simulink library "AEMS_Standard_Library"  (R2016b)
settings: Solver=ode45  StartTime=0.0  StopTime=10.0  RelTol=1e-3
undefined symbols (not defined in the file or in its folder): BkPY, carto, Cbx_extegr, Cbx_lpegrsys, Cbx_portegr, Cnx_bnk_nr_conf, Cnx_cyl_nr_conf, ConfigManagement, configuration_management, Cxx_dcm_io_tmr_end_xxxx, Cxx_dcm_rt_tmr_end, Cxx_DID_xxxx_IO_max, Cxx_DID_xxxx_IO_min, Cxx_egrhsofs, Cxx_vmaniegi, DEM_DEBOUNCE_FREEZE, DEM_DTR_CTL_INVISIBLE, DEM_DTR_CTL_NORMAL, Dem_DtrId2_XXX, Dem_DtrId3_XXX, Dem_DtrId4_XXX, Dem_DtrId5_XXX, Dem_DtrId6_XXX, Dem_DtrId7_XXX, Dem_DtrId8_XXX, Dem_DtrId9_XXX, Dem_DtrId_XXX, Dem_EnableConditionId2_XXX, Dem_EnableConditionId3_XXX, Dem_EnableConditionId4_XXX, Dem_EnableConditionId5_XXX, Dem_EnableConditionId6_XXX, Dem_EnableConditionId7_XXX, Dem_EnableConditionId8_XXX, Dem_EnableConditionId_XXX, Dem_EventId, Dem_EventId2_XXX, Dem_EventId3_XXX, Dem_EventId4_XXX, Dem_EventId5_XXX, Dem_EventId6_XXX, Dem_EventId7_XXX, Dem_EventId8_XXX, Dem_EventId9_XXX, Dem_EventId_Device_Faulttype, Dem_EventId_XXX, DEM_IUMPR_GENERAL_DENOMINATOR, DEM_OPCYC_IGNITION, Dem_RatioId2_XXX, Dem_RatioId3_XXX, Dem_RatioId4_XXX, Dem_RatioId5_XXX, Dem_RatioId6_XXX, Dem_RatioId7_XXX, Dem_RatioId8_XXX, Dem_RatioId_XXX, Dem_StorageConditionId2_XXX, Dem_StorageConditionId3_XXX, Dem_StorageConditionId4_XXX, Dem_StorageConditionId5_XXX ... (+65)
libraries: AEMS_Standard_Library x477, simulink x2
(part 31 of 39)

== system AEMS_Standard_Library/SUB/AEMS_DEM_COUNTER_BASED_DEBOUNCE_THRSHOLD_DYN_8D/AEMS_DEM_COUNTER_BASED_DEBOUNCE_THRSHOLD_DYN_CALL7 ==
  conditionfulfilled : Inport
  prefailed : Inport  Port=2
  prepassed : Inport  Port=3
  DemDebounceBehavior : Inport  Port=4
  failedthreshold : Inport  Port=5
  DemCounterIncrementStepSize : Inport  Port=6
  DemCounterJumpUp : Inport  Port=7
  DemCounterJumpUpValue : Inport  Port=8
  passedthreshold : Inport  Port=9
  DemCounterDecrementStepSize : Inport  Port=10
  DemCounterJumpDown : Inport  Port=11
  DemCounterJumpDownValue : Inport  Port=12
  reseteventdebounce : Inport  Port=13
  Enable : EnablePort
      settings: AttributesFormatString=StatesWhenEnabling = %<StatesWhenEnabling>
  AEMS_DEM_COUNTERBASEDDEBOUNCE : AEMS_Standard_Library/SUB/AEMS_DEM_COUNTERBASEDDEBOUNCE  Tag=[LIB]  eventid=Dem_EventId_Device7_Faulttype
      settings: AttributesFormatString=|
      | %<MaskType>
      | EventId: %<eventid>
  debouncevalue : Outport
      settings: AttributesFormatString=<initial=%<InitialOutput>>\n<whendisabled=%<OutputWhenDisabled>>
  failed : Outport  Port=2
      settings: AttributesFormatString=<initial=%<InitialOutput>>\n<whendisabled=%<OutputWhenDisabled>>
  passed : Outport  Port=3
      settings: AttributesFormatString=<initial=%<InitialOutput>>\n<whendisabled=%<OutputWhenDisabled>>
  wires:
  DemCounterJumpDownValue/1 -> AEMS_DEM_COUNTERBASEDDEBOUNCE/13
  DemCounterDecrementStepSize/1 -> AEMS_DEM_COUNTERBASEDDEBOUNCE/11
  DemCounterJumpUp/1 -> AEMS_DEM_COUNTERBASEDDEBOUNCE/8
  DemCounterIncrementStepSize/1 -> AEMS_DEM_COUNTERBASEDDEBOUNCE/7
  DemDebounceBehavior/1 -> AEMS_DEM_COUNTERBASEDDEBOUNCE/5
  DemCounterJumpDown/1 -> AEMS_DEM_COUNTERBASEDDEBOUNCE/12
  failedthreshold/1 -> AEMS_DEM_COUNTERBASEDDEBOUNCE/6
  passedthreshold/1 -> AEMS_DEM_COUNTERBASEDDEBOUNCE/10
  DemCounterJumpUpValue/1 -> AEMS_DEM_COUNTERBASEDDEBOUNCE/9
  reseteventdebounce/1 -> AEMS_DEM_COUNTERBASEDDEBOUNCE/4
  AEMS_DEM_COUNTERBASEDDEBOUNCE/3 -> passed/1
  AEMS_DEM_COUNTERBASEDDEBOUNCE/2 -> failed/1
  AEMS_DEM_COUNTERBASEDDEBOUNCE/1 -> debouncevalue/1
  prefailed/1 -> AEMS_DEM_COUNTERBASEDDEBOUNCE/2
  prepassed/1 -> AEMS_DEM_COUNTERBASEDDEBOUNCE/3
  conditionfulfilled/1 -> AEMS_DEM_COUNTERBASEDDEBOUNCE/1

== system AEMS_Standard_Library/SUB/AEMS_DEM_COUNTER_BASED_DEBOUNCE_THRSHOLD_DYN_8D/AEMS_DEM_COUNTER_BASED_DEBOUNCE_THRSHOLD_DYN_CALL8 ==
  conditionfulfilled : Inport
  prefailed : Inport  Port=2
  prepassed : Inport  Port=3
  DemDebounceBehavior : Inport  Port=4
  failedthreshold : Inport  Port=5
  DemCounterIncrementStepSize : Inport  Port=6
  DemCounterJumpUp : Inport  Port=7
  DemCounterJumpUpValue : Inport  Port=8
  passedthreshold : Inport  Port=9
  DemCounterDecrementStepSize : Inport  Port=10
  DemCounterJumpDown : Inport  Port=11
  DemCounterJumpDownValue : Inport  Port=12
  reseteventdebounce : Inport  Port=13
  Enable : EnablePort
      settings: AttributesFormatString=StatesWhenEnabling = %<StatesWhenEnabling>
  AEMS_DEM_COUNTERBASEDDEBOUNCE : AEMS_Standard_Library/SUB/AEMS_DEM_COUNTERBASEDDEBOUNCE  Tag=[LIB]  eventid=Dem_EventId_Device8_Faulttype
      settings: AttributesFormatString=|
      | %<MaskType>
      | EventId: %<eventid>
  debouncevalue : Outport
      settings: AttributesFormatString=<initial=%<InitialOutput>>\n<whendisabled=%<OutputWhenDisabled>>
  failed : Outport  Port=2
      settings: AttributesFormatString=<initial=%<InitialOutput>>\n<whendisabled=%<OutputWhenDisabled>>
  passed : Outport  Port=3
      settings: AttributesFormatString=<initial=%<InitialOutput>>\n<whendisabled=%<OutputWhenDisabled>>
  wires:
  DemCounterJumpUp/1 -> AEMS_DEM_COUNTERBASEDDEBOUNCE/8
  failedthreshold/1 -> AEMS_DEM_COUNTERBASEDDEBOUNCE/6
  DemCounterJumpDown/1 -> AEMS_DEM_COUNTERBASEDDEBOUNCE/12
  passedthreshold/1 -> AEMS_DEM_COUNTERBASEDDEBOUNCE/10
  DemCounterIncrementStepSize/1 -> AEMS_DEM_COUNTERBASEDDEBOUNCE/7
  DemDebounceBehavior/1 -> AEMS_DEM_COUNTERBASEDDEBOUNCE/5
  DemCounterDecrementStepSize/1 -> AEMS_DEM_COUNTERBASEDDEBOUNCE/11
  DemCounterJumpDownValue/1 -> AEMS_DEM_COUNTERBASEDDEBOUNCE/13
  DemCounterJumpUpValue/1 -> AEMS_DEM_COUNTERBASEDDEBOUNCE/9
  reseteventdebounce/1 -> AEMS_DEM_COUNTERBASEDDEBOUNCE/4
  conditionfulfilled/1 -> AEMS_DEM_COUNTERBASEDDEBOUNCE/1
  prepassed/1 -> AEMS_DEM_COUNTERBASEDDEBOUNCE/3
  prefailed/1 -> AEMS_DEM_COUNTERBASEDDEBOUNCE/2
  AEMS_DEM_COUNTERBASEDDEBOUNCE/1 -> debouncevalue/1
  AEMS_DEM_COUNTERBASEDDEBOUNCE/2 -> failed/1
  AEMS_DEM_COUNTERBASEDDEBOUNCE/3 -> passed/1

== system AEMS_Standard_Library/SUB/AEMS_DEM_REP_IUMPR_1D/Dem_RepIUMPRDenLock_call1 ==
  denlock_call1 : EnablePort
      settings: AttributesFormatString=<states=%<StatesWhenEnabling>>
  AEMS_DEM_REPIUMPRDENLOCK1 : AEMS_Standard_Library/SUB/AEMS_DEM_REPIUMPRDENLOCK  Tag=[LIB]
      settings: AttributesFormatString=%<MaskType>
  RatioId_block1 : Constant  Value=Dem_RatioId_XXX  OutDataTypeStr=uint16
  wires:
  RatioId_block1/1 -> AEMS_DEM_REPIUMPRDENLOCK1/1  "ratioid"

== system AEMS_Standard_Library/SUB/AEMS_DEM_REP_IUMPR_1D/Dem_RepIUMPRDenRelease_call1 ==
  denrelease_call1 : EnablePort
      settings: AttributesFormatString=<states=%<StatesWhenEnabling>>
  AEMS_DEM_REPIUMPRDENRELEASE1 : AEMS_Standard_Library/SUB/AEMS_DEM_REPIUMPRDENRELEASE  Tag=[LIB]
      settings: AttributesFormatString=%<MaskType>
  RatioId_block1 : Constant  Value=Dem_RatioId_XXX  OutDataTypeStr=uint16
  wires:
  RatioId_block1/1 -> AEMS_DEM_REPIUMPRDENRELEASE1/1  "ratioid"

== system AEMS_Standard_Library/SUB/AEMS_DEM_REP_IUMPR_1D/Dem_RepIUMPRFaultDetect_call1 ==
  faultdetect_call1 : EnablePort
      settings: AttributesFormatString=<states=%<StatesWhenEnabling>>
  AEMS_DEM_REPIUMPRFAULTDETECT1 : AEMS_Standard_Library/SUB/AEMS_DEM_REPIUMPRFAULTDETECT  Tag=[LIB]
      settings: AttributesFormatString=%<MaskType>
  RatioId_block1 : Constant  Value=Dem_RatioId_XXX  OutDataTypeStr=uint16
  wires:
  RatioId_block1/1 -> AEMS_DEM_REPIUMPRFAULTDETECT1/1  "ratioid"

== system AEMS_Standard_Library/SUB/AEMS_DEM_REP_IUMPR_2D/Dem_RepIUMPRDenLock_Call1 ==
  denlock_call1 : EnablePort
      settings: AttributesFormatString=<states=%<StatesWhenEnabling>>
  AEMS_DEM_REPIUMPRDENLOCK1 : AEMS_Standard_Library/SUB/AEMS_DEM_REPIUMPRDENLOCK
      settings: AttributesFormatString=%<MaskType>
  RatioId_block1 : Constant  Value=Dem_RatioId_XXX  OutDataTypeStr=uint16
  wires:
  RatioId_block1/1 -> AEMS_DEM_REPIUMPRDENLOCK1/1  "ratioid1"

== system AEMS_Standard_Library/SUB/AEMS_DEM_REP_IUMPR_2D/Dem_RepIUMPRDenLock_Call2 ==
  denlock_call2 : EnablePort
      settings: AttributesFormatString=<states=%<StatesWhenEnabling>>
  AEMS_DEM_REPIUMPRDENLOCK2 : AEMS_Standard_Library/SUB/AEMS_DEM_REPIUMPRDENLOCK
      settings: AttributesFormatString=%<MaskType>
  RatioId_block2 : Constant  Value=Dem_RatioId2_XXX  OutDataTypeStr=uint16
  wires:
  RatioId_block2/1 -> AEMS_DEM_REPIUMPRDENLOCK2/1  "ratioid2"

== system AEMS_Standard_Library/SUB/AEMS_DEM_REP_IUMPR_2D/Dem_RepIUMPRDenRelease_Call1 ==
  denrelease_call1 : EnablePort
      settings: AttributesFormatString=<states=%<StatesWhenEnabling>>
  AEMS_DEM_REPIUMPRDENRELEASE1 : AEMS_Standard_Library/SUB/AEMS_DEM_REPIUMPRDENRELEASE
      settings: AttributesFormatString=%<MaskType>
  RatioId_block1 : Constant  Value=Dem_RatioId_XXX  OutDataTypeStr=uint16
  wires:
  RatioId_block1/1 -> AEMS_DEM_REPIUMPRDENRELEASE1/1  "ratioid1"

== system AEMS_Standard_Library/SUB/AEMS_DEM_REP_IUMPR_2D/Dem_RepIUMPRDenRelease_Call2 ==
  denrelease_call2 : EnablePort
      settings: AttributesFormatString=<states=%<StatesWhenEnabling>>
  AEMS_DEM_REPIUMPRDENRELEASE2 : AEMS_Standard_Library/SUB/AEMS_DEM_REPIUMPRDENRELEASE
      settings: AttributesFormatString=%<MaskType>
  RatioId_block2 : Constant  Value=Dem_RatioId2_XXX  OutDataTypeStr=uint16
  wires:
  RatioId_block2/1 -> AEMS_DEM_REPIUMPRDENRELEASE2/1  "ratioid2"

== system AEMS_Standard_Library/SUB/AEMS_DEM_REP_IUMPR_2D/Dem_RepIUMPRFaultDetect_Call1 ==
  faultdetect_call1 : EnablePort
      settings: AttributesFormatString=<states=%<StatesWhenEnabling>>
  AEMS_DEM_REPIUMPRFAULTDETECT1 : AEMS_Standard_Library/SUB/AEMS_DEM_REPIUMPRFAULTDETECT
      settings: AttributesFormatString=%<MaskType>
  RatioId_block1 : Constant  Value=Dem_RatioId_XXX  OutDataTypeStr=uint16
  wires:
  RatioId_block1/1 -> AEMS_DEM_REPIUMPRFAULTDETECT1/1  "ratioid1"

== system AEMS_Standard_Library/SUB/AEMS_DEM_REP_IUMPR_2D/Dem_RepIUMPRFaultDetect_Call2 ==
  faultdetect_call2 : EnablePort
      settings: AttributesFormatString=<states=%<StatesWhenEnabling>>
  AEMS_DEM_REPIUMPRFAULTDETECT2 : AEMS_Standard_Library/SUB/AEMS_DEM_REPIUMPRFAULTDETECT
      settings: AttributesFormatString=%<MaskType>
  RatioId_block2 : Constant  Value=Dem_RatioId2_XXX  OutDataTypeStr=uint16
  wires:
  RatioId_block2/1 -> AEMS_DEM_REPIUMPRFAULTDETECT2/1  "ratioid2"

== system AEMS_Standard_Library/SUB/AEMS_DEM_REP_IUMPR_8D/Dem_RepIUMPRDenLock_Call1 ==
  denlock_call1 : EnablePort
      settings: AttributesFormatString=<states=%<StatesWhenEnabling>>
  AEMS_DEM_REPIUMPRDENLOCK1 : AEMS_Standard_Library/SUB/AEMS_DEM_REPIUMPRDENLOCK  Tag=[LIB]
      settings: AttributesFormatString=%<MaskType>
  RatioId_block1 : Constant  Value=Dem_RatioId_XXX  OutDataTypeStr=uint16
  wires:
  RatioId_block1/1 -> AEMS_DEM_REPIUMPRDENLOCK1/1  "ratioid1"

== system AEMS_Standard_Library/SUB/AEMS_DEM_REP_IUMPR_8D/Dem_RepIUMPRDenLock_Call2 ==
  denlock_call2 : EnablePort
      settings: AttributesFormatString=<states=%<StatesWhenEnabling>>
  AEMS_DEM_REPIUMPRDENLOCK2 : AEMS_Standard_Library/SUB/AEMS_DEM_REPIUMPRDENLOCK  Tag=[LIB]
      settings: AttributesFormatString=%<MaskType>
  RatioId_block2 : Constant  Value=Dem_RatioId2_XXX  OutDataTypeStr=uint16
  wires:
  RatioId_block2/1 -> AEMS_DEM_REPIUMPRDENLOCK2/1  "ratioid2"

== system AEMS_Standard_Library/SUB/AEMS_DEM_REP_IUMPR_8D/Dem_RepIUMPRDenLock_Call3 ==
  denlock_call3 : EnablePort
      settings: AttributesFormatString=<states=%<StatesWhenEnabling>>
  AEMS_DEM_REPIUMPRDENLOCK3 : AEMS_Standard_Library/SUB/AEMS_DEM_REPIUMPRDENLOCK  Tag=[LIB]
      settings: AttributesFormatString=%<MaskType>
  RatioId_block3 : Constant  Value=Dem_RatioId3_XXX  OutDataTypeStr=uint16
  wires:
  RatioId_block3/1 -> AEMS_DEM_REPIUMPRDENLOCK3/1  "ratioid3"

== system AEMS_Standard_Library/SUB/AEMS_DEM_REP_IUMPR_8D/Dem_RepIUMPRDenLock_Call4 ==
  denlock_call4 : EnablePort
      settings: AttributesFormatString=<states=%<StatesWhenEnabling>>
  AEMS_DEM_REPIUMPRDENLOCK4 : AEMS_Standard_Library/SUB/AEMS_DEM_REPIUMPRDENLOCK  Tag=[LIB]
      settings: AttributesFormatString=%<MaskType>
  RatioId_block4 : Constant  Value=Dem_RatioId4_XXX  OutDataTypeStr=uint16
  wires:
  RatioId_block4/1 -> AEMS_DEM_REPIUMPRDENLOCK4/1  "ratioid4"

== system AEMS_Standard_Library/SUB/AEMS_DEM_REP_IUMPR_8D/Dem_RepIUMPRDenLock_Call5 ==
  denlock_call5 : EnablePort
      settings: AttributesFormatString=<states=%<StatesWhenEnabling>>
  AEMS_DEM_REPIUMPRDENLOCK5 : AEMS_Standard_Library/SUB/AEMS_DEM_REPIUMPRDENLOCK  Tag=[LIB]
      settings: AttributesFormatString=%<MaskType>
  RatioId_block5 : Constant  Value=Dem_RatioId5_XXX  OutDataTypeStr=uint16
  wires:
  RatioId_block5/1 -> AEMS_DEM_REPIUMPRDENLOCK5/1  "ratioid5"

== system AEMS_Standard_Library/SUB/AEMS_DEM_REP_IUMPR_8D/Dem_RepIUMPRDenLock_Call6 ==
  denlock_call6 : EnablePort
      settings: AttributesFormatString=<states=%<StatesWhenEnabling>>
  AEMS_DEM_REPIUMPRDENLOCK6 : AEMS_Standard_Library/SUB/AEMS_DEM_REPIUMPRDENLOCK  Tag=[LIB]
      settings: AttributesFormatString=%<MaskType>
  RatioId_block6 : Constant  Value=Dem_RatioId6_XXX  OutDataTypeStr=uint16
  wires:
  RatioId_block6/1 -> AEMS_DEM_REPIUMPRDENLOCK6/1  "ratioid6"

== system AEMS_Standard_Library/SUB/AEMS_DEM_REP_IUMPR_8D/Dem_RepIUMPRDenLock_Call7 ==
  denlock_call7 : EnablePort
      settings: AttributesFormatString=<states=%<StatesWhenEnabling>>
  AEMS_DEM_REPIUMPRDENLOCK7 : AEMS_Standard_Library/SUB/AEMS_DEM_REPIUMPRDENLOCK  Tag=[LIB]
      settings: AttributesFormatString=%<MaskType>
  RatioId_block7 : Constant  Value=Dem_RatioId7_XXX  OutDataTypeStr=uint16
  wires:
  RatioId_block7/1 -> AEMS_DEM_REPIUMPRDENLOCK7/1  "ratioid7"

== system AEMS_Standard_Library/SUB/AEMS_DEM_REP_IUMPR_8D/Dem_RepIUMPRDenLock_Call8 ==
  denlock_call8 : EnablePort
      settings: AttributesFormatString=<states=%<StatesWhenEnabling>>
  AEMS_DEM_REPIUMPRDENLOCK8 : AEMS_Standard_Library/SUB/AEMS_DEM_REPIUMPRDENLOCK  Tag=[LIB]
      settings: AttributesFormatString=%<MaskType>
  RatioId_block8 : Constant  Value=Dem_RatioId8_XXX  OutDataTypeStr=uint16
  wires:
  RatioId_block8/1 -> AEMS_DEM_REPIUMPRDENLOCK8/1  "ratioid8"

== system AEMS_Standard_Library/SUB/AEMS_DEM_REP_IUMPR_8D/Dem_RepIUMPRDenRelease_Call1 ==
  denrelease_call1 : EnablePort
      settings: AttributesFormatString=<states=%<StatesWhenEnabling>>
  AEMS_DEM_REPIUMPRDENRELEASE1 : AEMS_Standard_Library/SUB/AEMS_DEM_REPIUMPRDENRELEASE  Tag=[LIB]
      settings: AttributesFormatString=%<MaskType>
  RatioId_block1 : Constant  Value=Dem_RatioId_XXX  OutDataTypeStr=uint16
  wires:
  RatioId_block1/1 -> AEMS_DEM_REPIUMPRDENRELEASE1/1  "ratioid1"

== system AEMS_Standard_Library/SUB/AEMS_DEM_REP_IUMPR_8D/Dem_RepIUMPRDenRelease_Call2 ==
  denrelease_call2 : EnablePort
      settings: AttributesFormatString=<states=%<StatesWhenEnabling>>
  AEMS_DEM_REPIUMPRDENRELEASE2 : AEMS_Standard_Library/SUB/AEMS_DEM_REPIUMPRDENRELEASE  Tag=[LIB]
      settings: AttributesFormatString=%<MaskType>
  RatioId_block2 : Constant  Value=Dem_RatioId2_XXX  OutDataTypeStr=uint16
  wires:
  RatioId_block2/1 -> AEMS_DEM_REPIUMPRDENRELEASE2/1  "ratioid2"

== system AEMS_Standard_Library/SUB/AEMS_DEM_REP_IUMPR_8D/Dem_RepIUMPRDenRelease_Call3 ==
  denrelease_call3 : EnablePort
      settings: AttributesFormatString=<states=%<StatesWhenEnabling>>
  AEMS_DEM_REPIUMPRDENRELEASE3 : AEMS_Standard_Library/SUB/AEMS_DEM_REPIUMPRDENRELEASE  Tag=[LIB]
      settings: AttributesFormatString=%<MaskType>
  RatioId_block3 : Constant  Value=Dem_RatioId3_XXX  OutDataTypeStr=uint16
  wires:
  RatioId_block3/1 -> AEMS_DEM_REPIUMPRDENRELEASE3/1  "ratioid3"

== system AEMS_Standard_Library/SUB/AEMS_DEM_REP_IUMPR_8D/Dem_RepIUMPRDenRelease_Call4 ==
  denrelease_call4 : EnablePort
      settings: AttributesFormatString=<states=%<StatesWhenEnabling>>
  AEMS_DEM_REPIUMPRDENRELEASE4 : AEMS_Standard_Library/SUB/AEMS_DEM_REPIUMPRDENRELEASE  Tag=[LIB]
      settings: AttributesFormatString=%<MaskType>
  RatioId_block4 : Constant  Value=Dem_RatioId4_XXX  OutDataTypeStr=uint16
  wires:
  RatioId_block4/1 -> AEMS_DEM_REPIUMPRDENRELEASE4/1  "ratioid4"

== system AEMS_Standard_Library/SUB/AEMS_DEM_REP_IUMPR_8D/Dem_RepIUMPRDenRelease_Call5 ==
  denrelease_call5 : EnablePort
      settings: AttributesFormatString=<states=%<StatesWhenEnabling>>
  AEMS_DEM_REPIUMPRDENRELEASE5 : AEMS_Standard_Library/SUB/AEMS_DEM_REPIUMPRDENRELEASE  Tag=[LIB]
      settings: AttributesFormatString=%<MaskType>
  RatioId_block5 : Constant  Value=Dem_RatioId5_XXX  OutDataTypeStr=uint16
  wires:
  RatioId_block5/1 -> AEMS_DEM_REPIUMPRDENRELEASE5/1  "ratioid5"

== system AEMS_Standard_Library/SUB/AEMS_DEM_REP_IUMPR_8D/Dem_RepIUMPRDenRelease_Call6 ==
  denrelease_call6 : EnablePort
      settings: AttributesFormatString=<states=%<StatesWhenEnabling>>
  AEMS_DEM_REPIUMPRDENRELEASE6 : AEMS_Standard_Library/SUB/AEMS_DEM_REPIUMPRDENRELEASE  Tag=[LIB]
      settings: AttributesFormatString=%<MaskType>
  RatioId_block6 : Constant  Value=Dem_RatioId6_XXX  OutDataTypeStr=uint16
  wires:
  RatioId_block6/1 -> AEMS_DEM_REPIUMPRDENRELEASE6/1  "ratioid6"

== system AEMS_Standard_Library/SUB/AEMS_DEM_REP_IUMPR_8D/Dem_RepIUMPRDenRelease_Call7 ==
  denrelease_call7 : EnablePort
      settings: AttributesFormatString=<states=%<StatesWhenEnabling>>
  AEMS_DEM_REPIUMPRDENRELEASE7 : AEMS_Standard_Library/SUB/AEMS_DEM_REPIUMPRDENRELEASE  Tag=[LIB]
      settings: AttributesFormatString=%<MaskType>
  RatioId_block7 : Constant  Value=Dem_RatioId7_XXX  OutDataTypeStr=uint16
  wires:
  RatioId_block7/1 -> AEMS_DEM_REPIUMPRDENRELEASE7/1  "ratioid7"

== system AEMS_Standard_Library/SUB/AEMS_DEM_REP_IUMPR_8D/Dem_RepIUMPRDenRelease_Call8 ==
  denrelease_call8 : EnablePort
      settings: AttributesFormatString=<states=%<StatesWhenEnabling>>
  AEMS_DEM_REPIUMPRDENRELEASE8 : AEMS_Standard_Library/SUB/AEMS_DEM_REPIUMPRDENRELEASE  Tag=[LIB]
      settings: AttributesFormatString=%<MaskType>
  RatioId_block8 : Constant  Value=Dem_RatioId8_XXX  OutDataTypeStr=uint16
  wires:
  RatioId_block8/1 -> AEMS_DEM_REPIUMPRDENRELEASE8/1  "ratioid8"

== system AEMS_Standard_Library/SUB/AEMS_DEM_REP_IUMPR_8D/Dem_RepIUMPRFaultDetect_Call1 ==
  faultdetect_call1 : EnablePort
      settings: AttributesFormatString=<states=%<StatesWhenEnabling>>
  AEMS_DEM_REPIUMPRFAULTDETECT1 : AEMS_Standard_Library/SUB/AEMS_DEM_REPIUMPRFAULTDETECT  Tag=[LIB]
      settings: AttributesFormatString=%<MaskType>
  RatioId_block1 : Constant  Value=Dem_RatioId_XXX  OutDataTypeStr=uint16
  wires:
  RatioId_block1/1 -> AEMS_DEM_REPIUMPRFAULTDETECT1/1  "ratioid1"

== system AEMS_Standard_Library/SUB/AEMS_DEM_REP_IUMPR_8D/Dem_RepIUMPRFaultDetect_Call2 ==
  faultdetect_call2 : EnablePort
      settings: AttributesFormatString=<states=%<StatesWhenEnabling>>
  AEMS_DEM_REPIUMPRFAULTDETECT2 : AEMS_Standard_Library/SUB/AEMS_DEM_REPIUMPRFAULTDETECT  Tag=[LIB]
      settings: AttributesFormatString=%<MaskType>
  RatioId_block2 : Constant  Value=Dem_RatioId2_XXX  OutDataTypeStr=uint16
  wires:
  RatioId_block2/1 -> AEMS_DEM_REPIUMPRFAULTDETECT2/1  "ratioid2"

== system AEMS_Standard_Library/SUB/AEMS_DEM_REP_IUMPR_8D/Dem_RepIUMPRFaultDetect_Call3 ==
  faultdetect_call3 : EnablePort
      settings: AttributesFormatString=<states=%<StatesWhenEnabling>>
  AEMS_DEM_REPIUMPRFAULTDETECT3 : AEMS_Standard_Library/SUB/AEMS_DEM_REPIUMPRFAULTDETECT  Tag=[LIB]
      settings: AttributesFormatString=%<MaskType>
  RatioId_block3 : Constant  Value=Dem_RatioId3_XXX  OutDataTypeStr=uint16
  wires:
  RatioId_block3/1 -> AEMS_DEM_REPIUMPRFAULTDETECT3/1  "ratioid3"

== system AEMS_Standard_Library/SUB/AEMS_DEM_REP_IUMPR_8D/Dem_RepIUMPRFaultDetect_Call4 ==
  faultdetect_call4 : EnablePort
      settings: AttributesFormatString=<states=%<StatesWhenEnabling>>
  AEMS_DEM_REPIUMPRFAULTDETECT4 : AEMS_Standard_Library/SUB/AEMS_DEM_REPIUMPRFAULTDETECT  Tag=[LIB]
      settings: AttributesFormatString=%<MaskType>
  RatioId_block4 : Constant  Value=Dem_RatioId4_XXX  OutDataTypeStr=uint16
  wires:
  RatioId_block4/1 -> AEMS_DEM_REPIUMPRFAULTDETECT4/1  "ratioid4"

== system AEMS_Standard_Library/SUB/AEMS_DEM_REP_IUMPR_8D/Dem_RepIUMPRFaultDetect_Call5 ==
  faultdetect_call5 : EnablePort
      settings: AttributesFormatString=<states=%<StatesWhenEnabling>>
  AEMS_DEM_REPIUMPRFAULTDETECT5 : AEMS_Standard_Library/SUB/AEMS_DEM_REPIUMPRFAULTDETECT  Tag=[LIB]
      settings: AttributesFormatString=%<MaskType>
  RatioId_block5 : Constant  Value=Dem_RatioId5_XXX  OutDataTypeStr=uint16
  wires:
  RatioId_block5/1 -> AEMS_DEM_REPIUMPRFAULTDETECT5/1  "ratioid5"

== system AEMS_Standard_Library/SUB/AEMS_DEM_REP_IUMPR_8D/Dem_RepIUMPRFaultDetect_Call6 ==
  faultdetect_call6 : EnablePort
      settings: AttributesFormatString=<states=%<StatesWhenEnabling>>
  AEMS_DEM_REPIUMPRFAULTDETECT6 : AEMS_Standard_Library/SUB/AEMS_DEM_REPIUMPRFAULTDETECT  Tag=[LIB]
      settings: AttributesFormatString=%<MaskType>
  RatioId_block6 : Constant  Value=Dem_RatioId6_XXX  OutDataTypeStr=uint16
  wires:
  RatioId_block6/1 -> AEMS_DEM_REPIUMPRFAULTDETECT6/1  "ratioid6"

== system AEMS_Standard_Library/SUB/AEMS_DEM_REP_IUMPR_8D/Dem_RepIUMPRFaultDetect_Call7 ==
  faultdetect_call7 : EnablePort
      settings: AttributesFormatString=<states=%<StatesWhenEnabling>>
  AEMS_DEM_REPIUMPRFAULTDETECT7 : AEMS_Standard_Library/SUB/AEMS_DEM_REPIUMPRFAULTDETECT  Tag=[LIB]
      settings: AttributesFormatString=%<MaskType>
  RatioId_block7 : Constant  Value=Dem_RatioId7_XXX  OutDataTypeStr=uint16
  wires:
  RatioId_block7/1 -> AEMS_DEM_REPIUMPRFAULTDETECT7/1  "ratioid7"

== system AEMS_Standard_Library/SUB/AEMS_DEM_REP_IUMPR_8D/Dem_RepIUMPRFaultDetect_Call8 ==
  faultdetect_call8 : EnablePort
      settings: AttributesFormatString=<states=%<StatesWhenEnabling>>
  AEMS_DEM_REPIUMPRFAULTDETECT8 : AEMS_Standard_Library/SUB/AEMS_DEM_REPIUMPRFAULTDETECT  Tag=[LIB]
      settings: AttributesFormatString=%<MaskType>
  RatioId_block8 : Constant  Value=Dem_RatioId8_XXX  OutDataTypeStr=uint16
  wires:
  RatioId_block8/1 -> AEMS_DEM_REPIUMPRFAULTDETECT8/1  "ratioid8"

== system AEMS_Standard_Library/SUB/AEMS_DEM_REP_IUMPR_DEN_RELEASE_1D/Dem_RepIUMPRDenRelease_call ==
  denrelease_call : EnablePort
      settings: AttributesFormatString=<states=%<StatesWhenEnabling>>
  AEMS_DEM_REPIUMPRDENRELEASE : AEMS_Standard_Library/SUB/AEMS_DEM_REPIUMPRDENRELEASE  Tag=[LIB]
      settings: AttributesFormatString=%<MaskType>
  RatioId_block1 : Constant  Value=Dem_RatioId_XXX  OutDataTypeStr=uint16
  wires:
  RatioId_block1/1 -> AEMS_DEM_REPIUMPRDENRELEASE/1  "ratioid"

== system AEMS_Standard_Library/SUB/AEMS_DEM_REP_IUMPR_DEN_RELEASE_2D/Dem_RepIUMPRDenRelease_call1 ==
  denrelease_call1 : EnablePort
      settings: AttributesFormatString=<states=%<StatesWhenEnabling>>
  AEMS_DEM_REPIUMPRDENRELEASE : AEMS_Standard_Library/SUB/AEMS_DEM_REPIUMPRDENRELEASE  Tag=[LIB]
      settings: AttributesFormatString=%<MaskType>
  RatioId_block1 : Constant  Value=Dem_RatioId_XXX  OutDataTypeStr=uint16
  wires:
  RatioId_block1/1 -> AEMS_DEM_REPIUMPRDENRELEASE/1  "ratioid1"

== system AEMS_Standard_Library/SUB/AEMS_DEM_REP_IUMPR_DEN_RELEASE_2D/Dem_RepIUMPRDenRelease_call2 ==
  denrelease_call2 : EnablePort
      settings: AttributesFormatString=<states=%<StatesWhenEnabling>>
  AEMS_DEM_REPIUMPRDENRELEASE : AEMS_Standard_Library/SUB/AEMS_DEM_REPIUMPRDENRELEASE  Tag=[LIB]
      settings: AttributesFormatString=%<MaskType>
  RatioId_block2 : Constant  Value=Dem_RatioId2_XXX  OutDataTypeStr=uint16
  wires:
  RatioId_block2/1 -> AEMS_DEM_REPIUMPRDENRELEASE/1  "ratioid2"

== system AEMS_Standard_Library/SUB/AEMS_DEM_REP_IUMPR_DEN_RELEASE_8D/Dem_RepIUMPRDenRelease_call1 ==
  denrelease_call1 : EnablePort
      settings: AttributesFormatString=<states=%<StatesWhenEnabling>>
  AEMS_DEM_REPIUMPRDENRELEASE : AEMS_Standard_Library/SUB/AEMS_DEM_REPIUMPRDENRELEASE  Tag=[LIB]
      settings: AttributesFormatString=%<MaskType>
  RatioId_block1 : Constant  Value=Dem_RatioId_XXX  OutDataTypeStr=uint16
  wires:
  RatioId_block1/1 -> AEMS_DEM_REPIUMPRDENRELEASE/1  "ratioid1"

== system AEMS_Standard_Library/SUB/AEMS_DEM_REP_IUMPR_DEN_RELEASE_8D/Dem_RepIUMPRDenRelease_call2 ==
  denrelease_call2 : EnablePort
      settings: AttributesFormatString=<states=%<StatesWhenEnabling>>
  AEMS_DEM_REPIUMPRDENRELEASE : AEMS_Standard_Library/SUB/AEMS_DEM_REPIUMPRDENRELEASE  Tag=[LIB]
      settings: AttributesFormatString=%<MaskType>
  RatioId_block2 : Constant  Value=Dem_RatioId2_XXX  OutDataTypeStr=uint16
  wires:
  RatioId_block2/1 -> AEMS_DEM_REPIUMPRDENRELEASE/1  "ratioid2"

== system AEMS_Standard_Library/SUB/AEMS_DEM_REP_IUMPR_DEN_RELEASE_8D/Dem_RepIUMPRDenRelease_call3 ==
  denrelease_call3 : EnablePort
      settings: AttributesFormatString=<states=%<StatesWhenEnabling>>
  AEMS_DEM_REPIUMPRDENRELEASE : AEMS_Standard_Library/SUB/AEMS_DEM_REPIUMPRDENRELEASE  Tag=[LIB]
      settings: AttributesFormatString=%<MaskType>
  RatioId_block3 : Constant  Value=Dem_RatioId3_XXX  OutDataTypeStr=uint16
  wires:
  RatioId_block3/1 -> AEMS_DEM_REPIUMPRDENRELEASE/1  "ratioid3"

== system AEMS_Standard_Library/SUB/AEMS_DEM_REP_IUMPR_DEN_RELEASE_8D/Dem_RepIUMPRDenRelease_call4 ==
  denrelease_call4 : EnablePort
      settings: AttributesFormatString=<states=%<StatesWhenEnabling>>
  AEMS_DEM_REPIUMPRDENRELEASE : AEMS_Standard_Library/SUB/AEMS_DEM_REPIUMPRDENRELEASE  Tag=[LIB]
      settings: AttributesFormatString=%<MaskType>
  RatioId_block4 : Constant  Value=Dem_RatioId4_XXX  OutDataTypeStr=uint16
  wires:
  RatioId_block4/1 -> AEMS_DEM_REPIUMPRDENRELEASE/1  "ratioid4"

== system AEMS_Standard_Library/SUB/AEMS_DEM_REP_IUMPR_DEN_RELEASE_8D/Dem_RepIUMPRDenRelease_call5 ==
  denrelease_call5 : EnablePort
      settings: AttributesFormatString=<states=%<StatesWhenEnabling>>
  AEMS_DEM_REPIUMPRDENRELEASE : AEMS_Standard_Library/SUB/AEMS_DEM_REPIUMPRDENRELEASE  Tag=[LIB]
      settings: AttributesFormatString=%<MaskType>
  RatioId_block5 : Constant  Value=Dem_RatioId5_XXX  OutDataTypeStr=uint16
  wires:
  RatioId_block5/1 -> AEMS_DEM_REPIUMPRDENRELEASE/1  "ratioid5"

== system AEMS_Standard_Library/SUB/AEMS_DEM_REP_IUMPR_DEN_RELEASE_8D/Dem_RepIUMPRDenRelease_call6 ==
  denrelease_call6 : EnablePort
      settings: AttributesFormatString=<states=%<StatesWhenEnabling>>
  AEMS_DEM_REPIUMPRDENRELEASE : AEMS_Standard_Library/SUB/AEMS_DEM_REPIUMPRDENRELEASE  Tag=[LIB]
      settings: AttributesFormatString=%<MaskType>
  RatioId_block6 : Constant  Value=Dem_RatioId6_XXX  OutDataTypeStr=uint16
  wires:
  RatioId_block6/1 -> AEMS_DEM_REPIUMPRDENRELEASE/1  "ratioid6"

== system AEMS_Standard_Library/SUB/AEMS_DEM_REP_IUMPR_DEN_RELEASE_8D/Dem_RepIUMPRDenRelease_call7 ==
  denrelease_call7 : EnablePort
      settings: AttributesFormatString=<states=%<StatesWhenEnabling>>
  AEMS_DEM_REPIUMPRDENRELEASE : AEMS_Standard_Library/SUB/AEMS_DEM_REPIUMPRDENRELEASE  Tag=[LIB]
      settings: AttributesFormatString=%<MaskType>
  RatioId_block7 : Constant  Value=Dem_RatioId7_XXX  OutDataTypeStr=uint16
  wires:
  RatioId_block7/1 -> AEMS_DEM_REPIUMPRDENRELEASE/1  "ratioid7"

== system AEMS_Standard_Library/SUB/AEMS_DEM_REP_IUMPR_DEN_RELEASE_8D/Dem_RepIUMPRDenRelease_call8 ==
  denrelease_call8 : EnablePort
      settings: AttributesFormatString=<states=%<StatesWhenEnabling>>
  AEMS_DEM_REPIUMPRDENRELEASE : AEMS_Standard_Library/SUB/AEMS_DEM_REPIUMPRDENRELEASE  Tag=[LIB]
      settings: AttributesFormatString=%<MaskType>
  RatioId_block8 : Constant  Value=Dem_RatioId8_XXX  OutDataTypeStr=uint16
  wires:
  RatioId_block8/1 -> AEMS_DEM_REPIUMPRDENRELEASE/1  "ratioid8"

== system AEMS_Standard_Library/SUB/AEMS_DEM_REP_IUMPR_FAULTDETECT_1D/Dem_RepIUMPRFaultDetect_call1 ==
  faultdetect_call1 : EnablePort
      settings: AttributesFormatString=<states=%<StatesWhenEnabling>>
  AEMS_DEM_REPIUMPRFAULTDETECT1 : AEMS_Standard_Library/SUB/AEMS_DEM_REPIUMPRFAULTDETECT  Tag=[LIB]
      settings: AttributesFormatString=%<MaskType>
  RatioId_block1 : Constant  Value=Dem_RatioId_XXX  OutDataTypeStr=uint16
  wires:
  RatioId_block1/1 -> AEMS_DEM_REPIUMPRFAULTDETECT1/1  "ratioid"

== system AEMS_Standard_Library/SUB/AEMS_DEM_REP_IUMPR_FAULTDETECT_2D/Dem_RepIUMPRFaultDetect_Call1 ==
  faultdetect_call1 : EnablePort
      settings: AttributesFormatString=<states=%<StatesWhenEnabling>>
  AEMS_DEM_REPIUMPRFAULTDETECT1 : AEMS_Standard_Library/SUB/AEMS_DEM_REPIUMPRFAULTDETECT
      settings: AttributesFormatString=%<MaskType>
  RatioId_block1 : Constant  Value=Dem_RatioId_XXX  OutDataTypeStr=uint16
  wires:
  RatioId_block1/1 -> AEMS_DEM_REPIUMPRFAULTDETECT1/1  "ratioid1"

== system AEMS_Standard_Library/SUB/AEMS_DEM_REP_IUMPR_FAULTDETECT_2D/Dem_RepIUMPRFaultDetect_Call2 ==
  faultdetect_call2 : EnablePort
      settings: AttributesFormatString=<states=%<StatesWhenEnabling>>
  AEMS_DEM_REPIUMPRFAULTDETECT2 : AEMS_Standard_Library/SUB/AEMS_DEM_REPIUMPRFAULTDETECT
      settings: AttributesFormatString=%<MaskType>
  RatioId_block2 : Constant  Value=Dem_RatioId2_XXX  OutDataTypeStr=uint16
  wires:
  RatioId_block2/1 -> AEMS_DEM_REPIUMPRFAULTDETECT2/1  "ratioid2"

== system AEMS_Standard_Library/SUB/AEMS_DEM_REP_IUMPR_FAULTDETECT_8D/Dem_RepIUMPRFaultDetect_Call1 ==
  faultdetect_call1 : EnablePort
      settings: AttributesFormatString=<states=%<StatesWhenEnabling>>
  AEMS_DEM_REPIUMPRFAULTDETECT1 : AEMS_Standard_Library/SUB/AEMS_DEM_REPIUMPRFAULTDETECT  Tag=[LIB]
      settings: AttributesFormatString=%<MaskType>
  RatioId_block1 : Constant  Value=Dem_RatioId_XXX  OutDataTypeStr=uint16
  wires:
  RatioId_block1/1 -> AEMS_DEM_REPIUMPRFAULTDETECT1/1  "ratioid1"

== system AEMS_Standard_Library/SUB/AEMS_DEM_REP_IUMPR_FAULTDETECT_8D/Dem_RepIUMPRFaultDetect_Call2 ==
  faultdetect_call2 : EnablePort
      settings: AttributesFormatString=<states=%<StatesWhenEnabling>>
  AEMS_DEM_REPIUMPRFAULTDETECT2 : AEMS_Standard_Library/SUB/AEMS_DEM_REPIUMPRFAULTDETECT  Tag=[LIB]
      settings: AttributesFormatString=%<MaskType>
  RatioId_block2 : Constant  Value=Dem_RatioId2_XXX  OutDataTypeStr=uint16
  wires:
  RatioId_block2/1 -> AEMS_DEM_REPIUMPRFAULTDETECT2/1  "ratioid2"

== system AEMS_Standard_Library/SUB/AEMS_DEM_REP_IUMPR_FAULTDETECT_8D/Dem_RepIUMPRFaultDetect_Call3 ==
  faultdetect_call3 : EnablePort
      settings: AttributesFormatString=<states=%<StatesWhenEnabling>>
  AEMS_DEM_REPIUMPRFAULTDETECT3 : AEMS_Standard_Library/SUB/AEMS_DEM_REPIUMPRFAULTDETECT  Tag=[LIB]
      settings: AttributesFormatString=%<MaskType>
  RatioId_block3 : Constant  Value=Dem_RatioId3_XXX  OutDataTypeStr=uint16
  wires:
  RatioId_block3/1 -> AEMS_DEM_REPIUMPRFAULTDETECT3/1  "ratioid3"

== system AEMS_Standard_Library/SUB/AEMS_DEM_REP_IUMPR_FAULTDETECT_8D/Dem_RepIUMPRFaultDetect_Call4 ==
  faultdetect_call4 : EnablePort
      settings: AttributesFormatString=<states=%<StatesWhenEnabling>>
  AEMS_DEM_REPIUMPRFAULTDETECT4 : AEMS_Standard_Library/SUB/AEMS_DEM_REPIUMPRFAULTDETECT  Tag=[LIB]
      settings: AttributesFormatString=%<MaskType>
  RatioId_block4 : Constant  Value=Dem_RatioId4_XXX  OutDataTypeStr=uint16
  wires:
  RatioId_block4/1 -> AEMS_DEM_REPIUMPRFAULTDETECT4/1  "ratioid4"

== system AEMS_Standard_Library/SUB/AEMS_DEM_REP_IUMPR_FAULTDETECT_8D/Dem_RepIUMPRFaultDetect_Call5 ==
  faultdetect_call5 : EnablePort
      settings: AttributesFormatString=<states=%<StatesWhenEnabling>>
  AEMS_DEM_REPIUMPRFAULTDETECT5 : AEMS_Standard_Library/SUB/AEMS_DEM_REPIUMPRFAULTDETECT  Tag=[LIB]
      settings: AttributesFormatString=%<MaskType>
  RatioId_block5 : Constant  Value=Dem_RatioId5_XXX  OutDataTypeStr=uint16
  wires:
  RatioId_block5/1 -> AEMS_DEM_REPIUMPRFAULTDETECT5/1  "ratioid5"

== system AEMS_Standard_Library/SUB/AEMS_DEM_REP_IUMPR_FAULTDETECT_8D/Dem_RepIUMPRFaultDetect_Call6 ==
  faultdetect_call6 : EnablePort
      settings: AttributesFormatString=<states=%<StatesWhenEnabling>>
  AEMS_DEM_REPIUMPRFAULTDETECT6 : AEMS_Standard_Library/SUB/AEMS_DEM_REPIUMPRFAULTDETECT  Tag=[LIB]
      settings: AttributesFormatString=%<MaskType>
  RatioId_block6 : Constant  Value=Dem_RatioId6_XXX  OutDataTypeStr=uint16
  wires:
  RatioId_block6/1 -> AEMS_DEM_REPIUMPRFAULTDETECT6/1  "ratioid6"

== system AEMS_Standard_Library/SUB/AEMS_DEM_REP_IUMPR_FAULTDETECT_8D/Dem_RepIUMPRFaultDetect_Call7 ==
  faultdetect_call7 : EnablePort
      settings: AttributesFormatString=<states=%<StatesWhenEnabling>>
  AEMS_DEM_REPIUMPRFAULTDETECT7 : AEMS_Standard_Library/SUB/AEMS_DEM_REPIUMPRFAULTDETECT  Tag=[LIB]
      settings: AttributesFormatString=%<MaskType>
  RatioId_block7 : Constant  Value=Dem_RatioId7_XXX  OutDataTypeStr=uint16
  wires:
  RatioId_block7/1 -> AEMS_DEM_REPIUMPRFAULTDETECT7/1  "ratioid7"

== system AEMS_Standard_Library/SUB/AEMS_DEM_REP_IUMPR_FAULTDETECT_8D/Dem_RepIUMPRFaultDetect_Call8 ==
  faultdetect_call8 : EnablePort
      settings: AttributesFormatString=<states=%<StatesWhenEnabling>>
  AEMS_DEM_REPIUMPRFAULTDETECT8 : AEMS_Standard_Library/SUB/AEMS_DEM_REPIUMPRFAULTDETECT  Tag=[LIB]
      settings: AttributesFormatString=%<MaskType>
  RatioId_block8 : Constant  Value=Dem_RatioId8_XXX  OutDataTypeStr=uint16
  wires:
  RatioId_block8/1 -> AEMS_DEM_REPIUMPRFAULTDETECT8/1  "ratioid8"

== system AEMS_Standard_Library/SUB/AEMS_DEM_SET_DTR_1DS/Dem_SetDTR_Call ==
  customresult : Inport  Interpolate=off
  lowerlimit : Inport  Port=2  Interpolate=off
  upperlimit : Inport  Port=3  Interpolate=off
  ctrl_flag : Inport  Port=4  Interpolate=off
  set_flag : EnablePort
      settings: AttributesFormatString=<states=%<StatesWhenEnabling>>
  AEMS_DEM_SETDTR : AEMS_Standard_Library/SUB/AEMS_DEM_SETDTR  Tag=[LIB]
      settings: AttributesFormatString=%<MaskType>
  Ctrlval_block : Constant  Value=DEM_DTR_CTL_NORMAL  OutDataTypeStr=uint8
  Ctrlval_block1 : Constant  Value=DEM_DTR_CTL_INVISIBLE  OutDataTypeStr=uint8
  DTRId_block : Constant  Value=Dem_DtrId_XXX  OutDataTypeStr=uint16
  Data Type Conversion : DataTypeConversion  OutDataTypeStr=int32  SaturateOnIntegerOverflow=on
  Data Type Conversion1 : DataTypeConversion  OutDataTypeStr=int32  SaturateOnIntegerOverflow=on
  Data Type Conversion2 : DataTypeConversion  OutDataTypeStr=int32  SaturateOnIntegerOverflow=on
  Divide1 : Product  Inputs=*/  OutDataTypeStr=Inherit: Inherit via back propagation  SaturateOnIntegerOverflow=on
  Divide2 : Product  Inputs=*/  OutDataTypeStr=Inherit: Inherit via back propagation  SaturateOnIntegerOverflow=on
  Divide3 : Product  Inputs=*/  OutDataTypeStr=Inherit: Inherit via back propagation  SaturateOnIntegerOverflow=on
  Limitter1 : Saturate  UpperLimit=65535  LowerLimit=0
      settings: AttributesFormatString=<limits=%<UpperLimit>/%<LowerLimit>>
  Limitter2 : Saturate  UpperLimit=65535  LowerLimit=0
      settings: AttributesFormatString=<limits=%<UpperLimit>/%<LowerLimit>>
  Limitter3 : Saturate  UpperLimit=65535  LowerLimit=0
      settings: AttributesFormatString=<limits=%<UpperLimit>/%<LowerLimit>>
  Resolution_block1 : Constant  OutDataTypeStr=single
  Resolution_block2 : Constant  OutDataTypeStr=single
  Resolution_block3 : Constant  OutDataTypeStr=single
  Switch : Switch  Criteria=u2 ~= 0  ZeroCross=off  InputSameDT=on
      settings: AttributesFormatString=Criteria=%<Criteria>
  wires:
  Ctrlval_block1/1 -> Switch/3
  ctrl_flag/1 -> Switch/2
  Ctrlval_block/1 -> Switch/1
  Switch/1 -> AEMS_DEM_SETDTR/5  "ctrlval"
  DTRId_block/1 -> AEMS_DEM_SETDTR/1  "dtrid"
  Resolution_block1/1 -> Divide1/2
  Limitter1/1 -> Divide1/1
  Divide1/1 -> Data Type Conversion/1
  Divide2/1 -> Data Type Conversion1/1
  Limitter3/1 -> Divide3/1
  customresult/1 -> Limitter1/1
  lowerlimit/1 -> Limitter2/1
  upperlimit/1 -> Limitter3/1
  Divide3/1 -> Data Type Conversion2/1
  Data Type Conversion1/1 -> AEMS_DEM_SETDTR/3  "lowlimit"
  Data Type Conversion2/1 -> AEMS_DEM_SETDTR/4  "uplimit"
  Data Type Conversion/1 -> AEMS_DEM_SETDTR/2  "result"
  Limitter2/1 -> Divide2/1
  Resolution_block2/1 -> Divide2/2
  Resolution_block3/1 -> Divide3/2

== system AEMS_Standard_Library/SUB/AEMS_DEM_SET_DTR_1DS/deadzone ==
  testresult : Inport  Interpolate=off
  lowerlimit : Inport  Port=2  Interpolate=off
  upperlimit : Inport  Port=3  Interpolate=off
  Sum1 : Sum  Inputs=-+  OutDataTypeStr=Inherit: Inherit via back propagation  InputSameDT=on
  Sum3 : Sum  OutDataTypeStr=Inherit: Inherit via back propagation  SaturateOnIntegerOverflow=on  InputSameDT=on
  Switch{,1,3..4} (4 alike) : Switch  Criteria=u2 ~= 0  ZeroCross=off  InputSameDT=on
      settings: AttributesFormatString=Criteria=%<Criteria>
  relational2 : RelationalOperator  DisableCoverage=on  OutDataTypeStr=boolean  ZeroCross=off  RndMeth=Nearest  InputSameDT=on
  relational3 : RelationalOperator  DisableCoverage=on  Operator=<  OutDataTypeStr=boolean  ZeroCross=off  RndMeth=Nearest  InputSameDT=on
  relational4 : RelationalOperator  DisableCoverage=on  OutDataTypeStr=boolean  ZeroCross=off  RndMeth=Nearest  InputSameDT=on
  relational5 : RelationalOperator  DisableCoverage=on  Operator=<=  OutDataTypeStr=boolean  ZeroCross=off  RndMeth=Nearest  InputSameDT=on
  resolution_block1 : Constant  OutDataTypeStr=single
  resolution_block2 : Constant  OutDataTypeStr=single
  customresult : Outport
  wires:
  Switch/1 -> customresult/1  "customresult"
  Sum3/1 -> Switch1/1, relational2/2
  Switch4/1 -> Switch3/3
  Switch1/1 -> Switch/3
  lowerlimit/1 -> relational4/2, Sum1/2
  relational5/1 -> Switch4/2
  relational4/1 -> Switch3/2
  relational3/1 -> Switch1/2
  resolution_block1/1 -> Sum3/2
  upperlimit/1 -> Sum3/1, relational3/1
  relational2/1 -> Switch/2
  testresult/1 -> Switch/1, relational2/1, relational4/1, Switch3/1, Switch4/3, relational5/2, relational3/2
  Switch3/1 -> Switch1/3
  Sum1/1 -> relational5/1, Switch4/1
  resolution_block2/1 -> Sum1/1

== system AEMS_Standard_Library/SUB/AEMS_DEM_SET_DTR_1DU/Dem_SetDTR_Call ==
  testresult : Inport  Interpolate=off
  lowerlimit : Inport  Port=2  Interpolate=off
  upperlimit : Inport  Port=3  Interpolate=off
  ctrl_flag : Inport  Port=4  Interpolate=off
  set_flag : EnablePort
      settings: AttributesFormatString=<states=%<StatesWhenEnabling>>
  AEMS_DEM_SETDTR : AEMS_Standard_Library/SUB/AEMS_DEM_SETDTR
      settings: AttributesFormatString=%<MaskType>
  Ctrlval_block : Constant  Value=DEM_DTR_CTL_NORMAL  OutDataTypeStr=uint8
  Ctrlval_block1 : Constant  Value=DEM_DTR_CTL_INVISIBLE  OutDataTypeStr=uint8
  DTRId_block : Constant  Value=Dem_DtrId_XXX  OutDataTypeStr=uint16
  Data Type Conversion : DataTypeConversion  OutDataTypeStr=int32  SaturateOnIntegerOverflow=on
  Data Type Conversion1 : DataTypeConversion  OutDataTypeStr=int32  SaturateOnIntegerOverflow=on
  Data Type Conversion2 : DataTypeConversion  OutDataTypeStr=int32  SaturateOnIntegerOverflow=on
  Limitter1 : Saturate  UpperLimit=1  LowerLimit=0
      settings: AttributesFormatString=<limits=%<UpperLimit>/%<LowerLimit>>
  Limitter2 : Saturate  UpperLimit=1  LowerLimit=0
      settings: AttributesFormatString=<limits=%<UpperLimit>/%<LowerLimit>>
  Limitter3 : Saturate  UpperLimit=1  LowerLimit=0
      settings: AttributesFormatString=<limits=%<UpperLimit>/%<LowerLimit>>
  Sum : Sum  SaturateOnIntegerOverflow=on  InputSameDT=on
  Sum1 : Sum  SaturateOnIntegerOverflow=on  InputSameDT=on
  Sum2 : Sum  SaturateOnIntegerOverflow=on  InputSameDT=on
  Switch : Switch  Criteria=u2 ~= 0  ZeroCross=off  InputSameDT=on
      settings: AttributesFormatString=Criteria=%<Criteria>
  offset1 : Constant  Value=0  OutDataTypeStr=uint16
  offset2 : Constant  Value=0  OutDataTypeStr=uint16
  offset3 : Constant  Value=0  OutDataTypeStr=uint16
  wires:
  Data Type Conversion2/1 -> AEMS_DEM_SETDTR/4  "uplimit"
  Data Type Conversion1/1 -> AEMS_DEM_SETDTR/3  "lowlimit"
  Data Type Conversion/1 -> AEMS_DEM_SETDTR/2  "result"
  upperlimit/1 -> Limitter3/1
  lowerlimit/1 -> Limitter2/1
  testresult/1 -> Limitter1/1
  Sum2/1 -> Data Type Conversion2/1
  Sum1/1 -> Data Type Conversion1/1
  Sum/1 -> Data Type Conversion/1
  Limitter3/1 -> Sum2/2
  offset3/1 -> Sum2/1
  Limitter2/1 -> Sum1/2
  offset2/1 -> Sum1/1
  Limitter1/1 -> Sum/2
  offset1/1 -> Sum/1
  Ctrlval_block/1 -> Switch/1
  DTRId_block/1 -> AEMS_DEM_SETDTR/1  "dtrid"
  Switch/1 -> AEMS_DEM_SETDTR/5  "ctrlval"
  Ctrlval_block1/1 -> Switch/3
  ctrl_flag/1 -> Switch/2  "ctrl_flag"

== system AEMS_Standard_Library/SUB/AEMS_DEM_SET_DTR_2DS/Deadzone ==
  testresult : Inport  Interpolate=off
  lowerlimit : Inport  Port=2  Interpolate=off
  upperlimit : Inport  Port=3  Interpolate=off
  Sum1 : Sum  Inputs=-+  OutDataTypeStr=Inherit: Inherit via back propagation  InputSameDT=on
  Sum3 : Sum  OutDataTypeStr=Inherit: Inherit via back propagation  SaturateOnIntegerOverflow=on  InputSameDT=on
  Switch{,1,3..4} (4 alike) : Switch  Criteria=u2 ~= 0  ZeroCross=off  InputSameDT=on
      settings: AttributesFormatString=Criteria=%<Criteria>
  relational2 : RelationalOperator  DisableCoverage=on  OutDataTypeStr=boolean  ZeroCross=off  RndMeth=Nearest  InputSameDT=on
  relational3 : RelationalOperator  DisableCoverage=on  Operator=<  OutDataTypeStr=boolean  ZeroCross=off  RndMeth=Nearest  InputSameDT=on
  relational4 : RelationalOperator  DisableCoverage=on  OutDataTypeStr=boolean  ZeroCross=off  RndMeth=Nearest  InputSameDT=on
  relational5 : RelationalOperator  DisableCoverage=on  Operator=<=  OutDataTypeStr=boolean  ZeroCross=off  RndMeth=Nearest  InputSameDT=on
  resolution_block1 : Constant  OutDataTypeStr=single
  resolution_block2 : Constant  OutDataTypeStr=single
  customresult : Outport
  wires:
  Switch/1 -> customresult/1  "customresult"
  Sum3/1 -> Switch1/1, relational2/2
  Switch4/1 -> Switch3/3
  Switch1/1 -> Switch/3
  lowerlimit/1 -> relational4/2, Sum1/2
  relational5/1 -> Switch4/2
  relational4/1 -> Switch3/2
  relational3/1 -> Switch1/2
  resolution_block1/1 -> Sum3/2
  upperlimit/1 -> Sum3/1, relational3/1
  relational2/1 -> Switch/2
  testresult/1 -> Switch/1, relational2/1, relational4/1, Switch3/1, Switch4/3, relational5/2, relational3/2
  Switch3/1 -> Switch1/3
  Sum1/1 -> relational5/1, Switch4/1
  resolution_block2/1 -> Sum1/1

== system AEMS_Standard_Library/SUB/AEMS_DEM_SET_DTR_2DS/Dem_SetDTR_Call1 ==
  customresult1 : Inport  Interpolate=off
  lowerlimit1 : Inport  Port=2  Interpolate=off
  upperlimit1 : Inport  Port=3  Interpolate=off
  ctrl_flag1 : Inport  Port=4  Interpolate=off
  set_flag1 : EnablePort
      settings: AttributesFormatString=<states=%<StatesWhenEnabling>>
  AEMS_DEM_SETDTR : AEMS_Standard_Library/SUB/AEMS_DEM_SETDTR
      settings: AttributesFormatString=%<MaskType>
  Ctrlval_block1 : Constant  Value=DEM_DTR_CTL_NORMAL  OutDataTypeStr=uint8
  Ctrlval_block2 : Constant  Value=DEM_DTR_CTL_INVISIBLE  OutDataTypeStr=uint8
  DTRId_block1 : Constant  Value=Dem_DtrId_XXX  OutDataTypeStr=uint16
  Data Type Conversion : DataTypeConversion  OutDataTypeStr=int32  SaturateOnIntegerOverflow=on
  Data Type Conversion1 : DataTypeConversion  OutDataTypeStr=int32  SaturateOnIntegerOverflow=on
  Data Type Conversion2 : DataTypeConversion  OutDataTypeStr=int32  SaturateOnIntegerOverflow=on
  Divide1 : Product  Inputs=*/  OutDataTypeStr=Inherit: Inherit via back propagation  SaturateOnIntegerOverflow=on
  Divide2 : Product  Inputs=*/  OutDataTypeStr=Inherit: Inherit via back propagation  SaturateOnIntegerOverflow=on
  Divide3 : Product  Inputs=*/  OutDataTypeStr=Inherit: Inherit via back propagation  SaturateOnIntegerOverflow=on
  Limitter1 : Saturate  UpperLimit=1  LowerLimit=0
      settings: AttributesFormatString=<limits=%<UpperLimit>/%<LowerLimit>>
  Limitter2 : Saturate  UpperLimit=1  LowerLimit=0
      settings: AttributesFormatString=<limits=%<UpperLimit>/%<LowerLimit>>
  Limitter3 : Saturate  UpperLimit=1  LowerLimit=0
      settings: AttributesFormatString=<limits=%<UpperLimit>/%<LowerLimit>>
  Resolution_block1 : Constant  OutDataTypeStr=single
  Resolution_block2 : Constant  OutDataTypeStr=single
  Resolution_block3 : Constant  OutDataTypeStr=single
  Switch : Switch  Criteria=u2 ~= 0  ZeroCross=off  InputSameDT=on
      settings: AttributesFormatString=Criteria=%<Criteria>
  wires:
  DTRId_block1/1 -> AEMS_DEM_SETDTR/1  "dtrid1"
  Resolution_block1/1 -> Divide1/2
  Limitter1/1 -> Divide1/1
  Divide1/1 -> Data Type Conversion/1
  Divide2/1 -> Data Type Conversion1/1
  Limitter3/1 -> Divide3/1
  customresult1/1 -> Limitter1/1
  lowerlimit1/1 -> Limitter2/1
  upperlimit1/1 -> Limitter3/1
  Divide3/1 -> Data Type Conversion2/1
  Data Type Conversion1/1 -> AEMS_DEM_SETDTR/3  "lowlimit1"
  Data Type Conversion2/1 -> AEMS_DEM_SETDTR/4  "uplimit1"
  Data Type Conversion/1 -> AEMS_DEM_SETDTR/2  "result1"
  Limitter2/1 -> Divide2/1
  Resolution_block2/1 -> Divide2/2
  Resolution_block3/1 -> Divide3/2
  Switch/1 -> AEMS_DEM_SETDTR/5  "ctrlval1"
  Ctrlval_block1/1 -> Switch/1
  ctrl_flag1/1 -> Switch/2
  Ctrlval_block2/1 -> Switch/3

== system AEMS_Standard_Library/SUB/AEMS_DEM_SET_DTR_2DS/Dem_SetDTR_Call2 ==
  customresult2 : Inport  Interpolate=off
  lowerlimit2 : Inport  Port=2  Interpolate=off
  upperlimit2 : Inport  Port=3  Interpolate=off
  ctrl_flag2 : Inport  Port=4  Interpolate=off
  set_flag2 : EnablePort
      settings: AttributesFormatString=<states=%<StatesWhenEnabling>>
  AEMS_DEM_SETDTR2 : AEMS_Standard_Library/SUB/AEMS_DEM_SETDTR
      settings: AttributesFormatString=%<MaskType>
  Ctrlval_block1 : Constant  Value=DEM_DTR_CTL_NORMAL  OutDataTypeStr=uint8
  Ctrlval_block2 : Constant  Value=DEM_DTR_CTL_INVISIBLE  OutDataTypeStr=uint8
  DTRId_block2 : Constant  Value=Dem_DtrId2_XXX  OutDataTypeStr=uint16
  Data Type Conversion : DataTypeConversion  OutDataTypeStr=int32  SaturateOnIntegerOverflow=on
  Data Type Conversion1 : DataTypeConversion  OutDataTypeStr=int32  SaturateOnIntegerOverflow=on
  Data Type Conversion2 : DataTypeConversion  OutDataTypeStr=int32  SaturateOnIntegerOverflow=on
  Divide1 : Product  Inputs=*/  OutDataTypeStr=Inherit: Inherit via back propagation  SaturateOnIntegerOverflow=on
  Divide2 : Product  Inputs=*/  OutDataTypeStr=Inherit: Inherit via back propagation  SaturateOnIntegerOverflow=on
  Divide3 : Product  Inputs=*/  OutDataTypeStr=Inherit: Inherit via back propagation  SaturateOnIntegerOverflow=on
  Limitter4 : Saturate  UpperLimit=1  LowerLimit=0
      settings: AttributesFormatString=<limits=%<UpperLimit>/%<LowerLimit>>
  Limitter5 : Saturate  UpperLimit=1  LowerLimit=0
      settings: AttributesFormatString=<limits=%<UpperLimit>/%<LowerLimit>>
  Limitter6 : Saturate  UpperLimit=1  LowerLimit=0
      settings: AttributesFormatString=<limits=%<UpperLimit>/%<LowerLimit>>
  Resolution_block4 : Constant  OutDataTypeStr=single
  Resolution_block5 : Constant  OutDataTypeStr=single
  Resolution_block6 : Constant  OutDataTypeStr=single
  Switch : Switch  Criteria=u2 ~= 0  ZeroCross=off  InputSameDT=on
      settings: AttributesFormatString=Criteria=%<Criteria>
  wires:
  DTRId_block2/1 -> AEMS_DEM_SETDTR2/1  "dtrid2"
  Resolution_block4/1 -> Divide1/2
  Limitter4/1 -> Divide1/1
  Limitter6/1 -> Divide3/1
  customresult2/1 -> Limitter4/1
  lowerlimit2/1 -> Limitter5/1
  upperlimit2/1 -> Limitter6/1
  Data Type Conversion1/1 -> AEMS_DEM_SETDTR2/3  "lowlimit2"
  Data Type Conversion2/1 -> AEMS_DEM_SETDTR2/4  "uplimit2"
  Data Type Conversion/1 -> AEMS_DEM_SETDTR2/2  "result2"
  Limitter5/1 -> Divide2/1
  Resolution_block5/1 -> Divide2/2
  Resolution_block6/1 -> Divide3/2
  Switch/1 -> AEMS_DEM_SETDTR2/5  "ctrlval2"
  Ctrlval_block1/1 -> Switch/1
  ctrl_flag2/1 -> Switch/2
  Ctrlval_block2/1 -> Switch/3
  Divide1/1 -> Data Type Conversion/1
  Divide2/1 -> Data Type Conversion1/1
  Divide3/1 -> Data Type Conversion2/1
